simulink model "Problem_2_4"  (R2018a)
settings: Solver=VariableStepAuto  StartTime=0.0  StopTime=10.0  RelTol=1e-3
undefined symbols (not defined in the file): b, ks, kt, M, m
settings Model: Creator=lasse  LastModifiedBy=pala

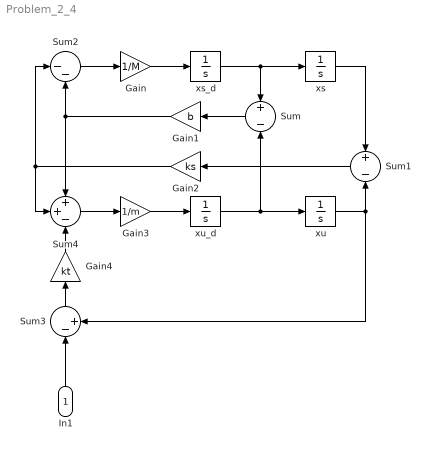
== system Problem_2_4 ==
  In1 : Inport
  Gain : Gain  Gain=1/M
  Gain1 : Gain  Gain=b
  Gain2 : Gain  Gain=ks
  Gain3 : Gain  Gain=1/m
  Gain4 : Gain  Gain=kt
  Sum : Sum  Inputs=+|-
  Sum1 : Sum  Inputs=+|-
  Sum2 : Sum  Inputs=|--
  Sum3 : Sum  Inputs=|-+
  Sum4 : Sum  Inputs=++-
  xs : Integrator
  xs_d : Integrator
  xu : Integrator
  xu_d : Integrator
  wires:
  Gain/1 -> xs_d/1
  xs_d/1 -> xs/1, Sum/1
  xu_d/1 -> xu/1, Sum/2
  Sum/1 -> Gain1/1
  xs/1 -> Sum1/1
  xu/1 -> Sum3/2, Sum1/2
  Sum1/1 -> Gain2/1
  Gain3/1 -> xu_d/1
  Sum2/1 -> Gain/1
  Gain1/1 -> Sum4/1, Sum2/2
  Gain2/1 -> Sum2/1, Sum4/2
  Sum4/1 -> Gain3/1
  In1/1 -> Sum3/1
  Gain4/1 -> Sum4/3
  Sum3/1 -> Gain4/1
